simulink model "FBL_WP4_sim"  (R2023b)
settings: Solver=VariableStepAuto  StartTime=0.0  StopTime=10.0  RelTol=1e-6
undefined symbols (not defined in the file): r
settings Model: Creator=giov_russo  LastModifiedBy=beniaminosquitieri
settings SolverCC: AlgebraicLoopSolver=TrustRegion
settings DebuggingCC: UnconnectedInputMsg=warning  UnconnectedOutputMsg=warning  UnconnectedLineMsg=warning
settings ModelReferenceCC: EnableRefExpFcnMdlSchedulingChecks=on

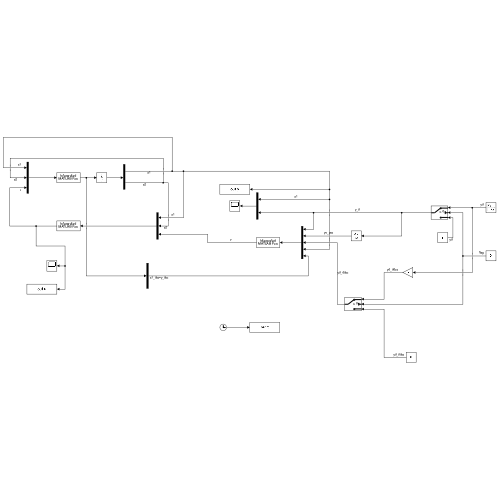
[thumbnail: Simulink's stored preview of the top-level diagram]
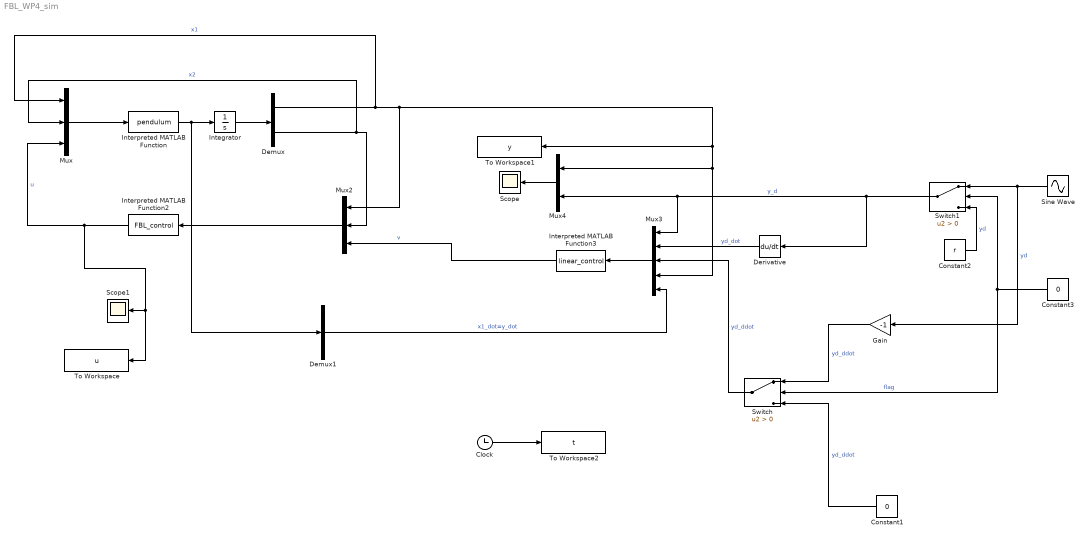
== system FBL_WP4_sim ==
  Clock : Clock
  Constant1 : Constant  Value=0
  Constant2 : Constant  Value=r
  Constant3 : Constant  Value=0
  Demux : Demux  Outputs=2
  Demux1 : Demux  Outputs=1
  Derivative : Derivative
  Gain : Gain  Gain=-1
  Integrator : Integrator
  Interpreted MATLAB Function : MATLABFcn  MATLABFcn=pendulum  OutputDimensions=2
  Interpreted MATLAB Function2 : MATLABFcn  MATLABFcn=FBL_control  OutputDimensions=1
  Interpreted MATLAB Function3 : MATLABFcn  MATLABFcn=linear_control  OutputDimensions=1
  Mux : Mux  Inputs=3
  Mux2 : Mux  Inputs=3
  Mux3 : Mux  Inputs=5
  Mux4 : Mux  Inputs=2
  Scope : Scope
  Scope1 : Scope
  Sine Wave : Sin  SampleTime=0
  Switch : Switch  Criteria=u2 > Threshold  SaturateOnIntegerOverflow=off  InputSameDT=off
  Switch1 : Switch  Criteria=u2 > Threshold  SaturateOnIntegerOverflow=off  InputSameDT=off
  To Workspace : ToWorkspace  VariableName=u  SaveFormat=Timeseries  SampleTime=-1
  To Workspace1 : ToWorkspace  VariableName=y  SaveFormat=Timeseries  SampleTime=-1
  To Workspace2 : ToWorkspace  VariableName=t  SaveFormat=Timeseries  SampleTime=-1
  wires:
  Mux/1 -> Interpreted MATLAB Function/1
  Interpreted MATLAB Function/1 -> Demux1/1, Integrator/1
  Integrator/1 -> Demux/1
  Demux/1 -> To Workspace1/1, Mux4/1, Mux3/4, Mux2/1, Mux/1  "x1"
  Demux/2 -> Mux2/2, Mux/2  "x2"
  Mux2/1 -> Interpreted MATLAB Function2/1
  Interpreted MATLAB Function2/1 -> To Workspace/1, Scope1/1, Mux/3  "u"
  Mux3/1 -> Interpreted MATLAB Function3/1
  Mux4/1 -> Scope/1
  Interpreted MATLAB Function3/1 -> Mux2/3  "v"
  Derivative/1 -> Mux3/2  "yd_dot"
  Demux1/1 -> Mux3/5  "x1_dot=y_dot"
  Clock/1 -> To Workspace2/1
  Sine Wave/1 -> Gain/1, Switch1/1  "yd"
  Constant2/1 -> Switch1/3  "yd"
  Switch1/1 -> Derivative/1, Mux3/1, Mux4/2  "y_d"
  Constant1/1 -> Switch/3  "yd_ddot"
  Gain/1 -> Switch/1  "yd_ddot"
  Constant3/1 -> Switch1/2, Switch/2  "flag"
  Switch/1 -> Mux3/3  "yd_ddot"
